simulink model "Teller_bank"  (R2018a)
settings: Solver=VariableStepAuto  StartTime=0.0  StopTime=60.0  RelTol=1e-3
undefined symbols (not defined in the file): m, n
settings Model: Creator=acer  LastModifiedBy=acer

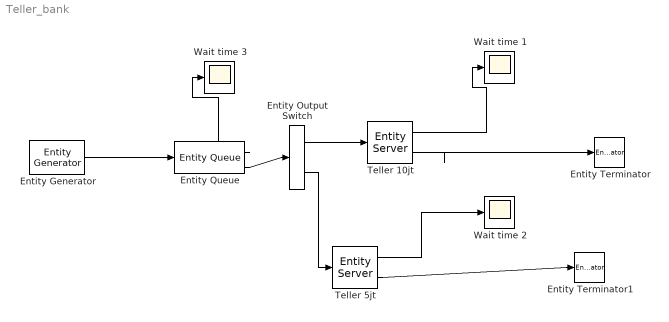
== system Teller_bank ==
  Entity Output Switch : EntityOutputSwitch  Priority=1  InputPortMessageModes=m  OutputPortMessageModes=m,m  SwitchAttributeName=Attribute1
  Entity Generator : EntityGenerator  OutputPortMessageModes=m  TimeSource=MATLAB action  IntergenerationTimeAction=|  GenerateAction=|  AttributeName=Attribute1|Attribute2  AttributeInitialValue=1|2  EntityType=Structured  EntityTypeName=Nasabah
      IntergenerationTimeAction=|
      | mean = 0.5;
      | dt = mean*rand();
      GenerateAction=|
      | persistent rngInit;
      | if isempty(rngInit)
      |     seed = 12345;
      |     rng(seed);
      |     rngInit = true;
      | end
      | 
      | % Pattern: Uniform distribution
      | % m: Minimum, M: Maximum
      | m = 1, M = 20;
      | x = m + (M - m) * rand;
  Entity Queue : EntityQueue  InputPortMessageModes=m  OutputPortMessageModes=n,m  Capacity=20  ExitAction=|  AverageWait=on
      | persistent rngInit;
      | if isempty(rngInit)
      |     seed = 12345;
      |     rng(seed);
      |     rngInit = true;
      | end
      | 
      | 
      | % Pattern: Uniform distribution
      | % m: Minimum, M: Maximum
      | m = 1, M = 10;
      | x1 = m + (M - m) * rand;
      settings: OutputPortMap=o2,o5
  Entity Terminator : EntityTerminator  InputPortMessageModes=m
  Entity Terminator1 : EntityTerminator  InputPortMessageModes=m
  "Teller 10jt " : EntityServer  InputPortMessageModes=m  OutputPortMessageModes=n,m  Capacity=1  ServiceTimeValue=3  ExitAction=|  NumberEntitiesDeparted=on
      | persistent rngInit;
      | if isempty(rngInit)
      |     seed = 12345;
      |     rng(seed);
      |     rngInit = true;
      | end
      | 
      | % Pattern: Uniform distribution
      | % m: Minimum, M: Maximum
      | m = 1, M = 10;
      | x = m + (M - m) * rand;
      settings: OutputPortMap=o0,o9
  "Teller 5jt " : EntityServer  InputPortMessageModes=m  OutputPortMessageModes=n,m  Capacity=1  ServiceTimeValue=2  NumberEntitiesDeparted=on
      settings: OutputPortMap=o0,o9
  Wait time 1 : Scope
  Wait time 2 : Scope
  Wait time 3 : Scope
  wires:
  "Teller 10jt "/2 -> Entity Terminator/1
  Entity Queue/2 -> Entity Output Switch/1
  Entity Output Switch/1 -> "Teller 10jt "/1
  Entity Output Switch/2 -> "Teller 5jt "/1
  "Teller 5jt "/2 -> Entity Terminator1/1
  Entity Generator/1 -> Entity Queue/1
  Entity Queue/1 -> Wait time 3/1
  "Teller 10jt "/1 -> Wait time 1/1
  "Teller 5jt "/1 -> Wait time 2/1
